simulink library "hmi"  (Simulink 8.1)
settings: Solver=ode1  StartTime=0.0  StopTime=Inf  FixedStep=0.001  RelTol=1e-3
PostLoadFcn:
  | , if any(exist('dsrtsu_mdlpostloadfcn', 'file') == [2, 3, 6]), try dsrtsu_mdlpostloadfcn('Execute', bdroot); catch fprintf('Error in PostLoadFcn (dsrtsu_mdlpostloadfcn) for model "%s":\n %s\n', bdroot, lasterr); end, end,
libraries: act x1, agg x1, brk x1, accs x1, ovr x1, otk x1, pkg x1, hcu_lib x1
settings Model: DSRTSU_INTERNAL_RTI_VER=450  DSRTSU_INTERNAL_RTI_TYPE=rti1401  RTICANMMDATA=struct('GeneralSetupData',struct('modelroot','D:\ELN150201_TAIWAN\trunk\AdasDragon\software\sw_development\arch\app\ifo','generalsettings',struct('filesettings',struct('destfolder',struct('Name','RTICANMM_FILES','Check',1),'buildfolder',struct('Name','.','Check',1),'AbsDestfolder',struct('Name','D:\ELN150201_TAIWAN\trunk\AdasDragon\software\sw_development\arch\app\ifo\RTICANMM_FILES'),'AbsBuildfolder',struct('Name','D:\ELN150201_TAIWAN\trunk\AdasDragon\software\sw_development\arch\app\ifo'))),'options',struct('addpaths',1,'rmpaths',1,'addtrcexclusion',logical(1),'cannavigator',struct('checkmonitoring',0),'show_usrtrc',0,'use_usrtrc',0),'advanced',struct('options',[1 1 1 1 1 1 1 1 1 1 1 1 1 1 1 1 1 1 1 1 1 1 1 1 1 1 1 1 1 1 1 1 1 1 1 1 1 1 1 1 1 1 1 1 1 1 1 1 1 1 1 1 1 1 1 1 1 1 1 1 1 1 1 1 1 1 1 1 1 1 1 1 1 1 1 1 1 1 1 1 1 1 1 1 1 1 1 1 1 1 1 1 1 1 1 1 1 1 1 1]),'MPSetup',{{}},'modelname','hmi','block','hmi'))  DSRTSU_INTERNAL_RTIFPGA=40  Creator=AT015411  LastModifiedBy=AT015555

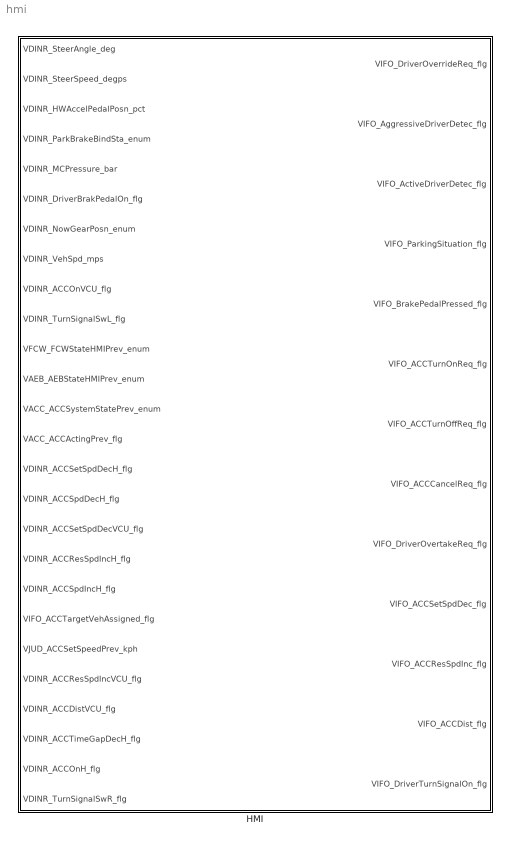
== system hmi ==
  HMI : Subsystem

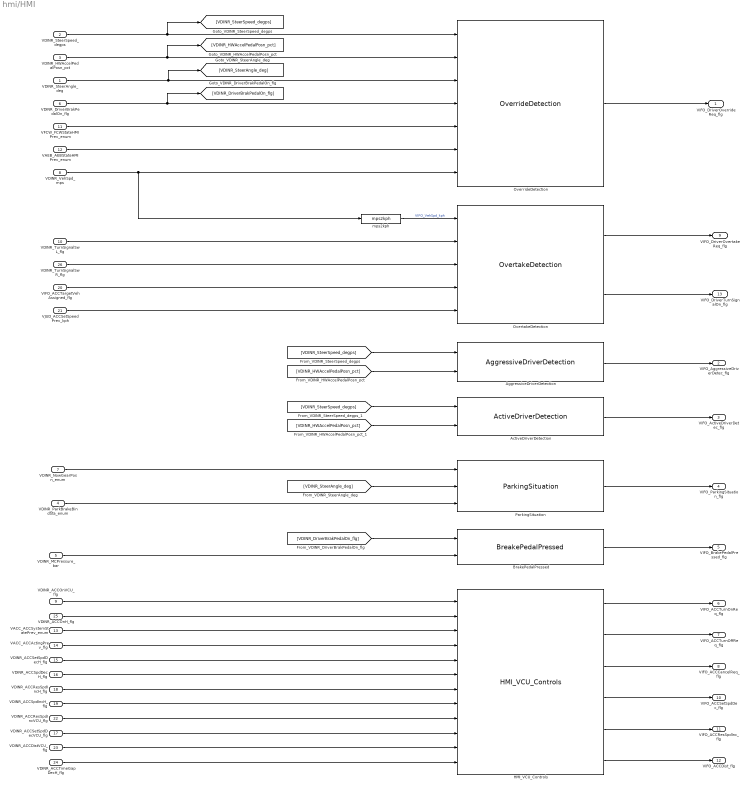
== system hmi/HMI ==
  VDINR_SteerAngle_deg : Inport
  VDINR_SteerSpeed_degps : Inport  Port=2
  VDINR_HWAccelPedalPosn_pct : Inport  Port=3
  VDINR_ParkBrakeBindSta_enum : Inport  Port=4
  VDINR_MCPressure_bar : Inport  Port=5
  VDINR_DriverBrakPedalOn_flg : Inport  Port=6
  VDINR_NowGearPosn_enum : Inport  Port=7
  VDINR_VehSpd_mps : Inport  Port=8
  VDINR_ACCOnVCU_flg : Inport  Port=9
  VDINR_TurnSignalSwL_flg : Inport  Port=10
  VFCW_FCWStateHMIPrev_enum : Inport  Port=11
  VAEB_AEBStateHMIPrev_enum : Inport  Port=12
  VACC_ACCSystemStatePrev_enum : Inport  Port=13
  VACC_ACCActingPrev_flg : Inport  Port=14
  VDINR_ACCSetSpdDecH_flg : Inport  Port=15
  VDINR_ACCSpdDecH_flg : Inport  Port=16
  VDINR_ACCSetSpdDecVCU_flg : Inport  Port=17
  VDINR_ACCResSpdIncH_flg : Inport  Port=18
  VDINR_ACCSpdIncH_flg : Inport  Port=19
  VIFO_ACCTargetVehAssigned_flg : Inport  Port=20
  VJUD_ACCSetSpeedPrev_kph : Inport  Port=21
  VDINR_ACCResSpdIncVCU_flg : Inport  Port=22
  VDINR_ACCDistVCU_flg : Inport  Port=23
  VDINR_ACCTimeGapDecH_flg : Inport  Port=24
  VDINR_ACCOnH_flg : Inport  Port=25
  VDINR_TurnSignalSwR_flg : Inport  Port=26
  ActiveDriverDetection : act/ActiveDriverDetection
  AggressiveDriverDetection : agg/AggressiveDriverDetection
  BrakePedalPressed : brk/BreakePedalPressed
  HMI_VCU_Controls : accs/HMI_VCU_Controls
  OverrideDetection : ovr/OverrideDetection
  OvertakeDetection : otk/OvertakeDetection
  ParkingSituation : pkg/ParkingSituation
  mps2kph : hcu_lib/mps2kph
  VIFO_DriverOverrideReq_flg : Outport
  VIFO_AggressiveDriverDetec_flg : Outport  Port=2
  VIFO_ActiveDriverDetec_flg : Outport  Port=3
  VIFO_ParkingSituation_flg : Outport  Port=4
  VIFO_BrakePedalPressed_flg : Outport  Port=5
  VIFO_ACCTurnOnReq_flg : Outport  Port=6
  VIFO_ACCTurnOffReq_flg : Outport  Port=7
  VIFO_ACCCancelReq_flg : Outport  Port=8
  VIFO_DriverOvertakeReq_flg : Outport  Port=9
  VIFO_ACCSetSpdDec_flg : Outport  Port=10
  VIFO_ACCResSpdInc_flg : Outport  Port=11
  VIFO_ACCDist_flg : Outport  Port=12
  VIFO_DriverTurnSignalOn_flg : Outport  Port=13
  wires:
  VDINR_ACCOnH_flg/1 -> HMI_VCU_Controls/2
  VDINR_ACCSpdIncH_flg/1 -> HMI_VCU_Controls/8
  VDINR_ACCSetSpdDecH_flg/1 -> HMI_VCU_Controls/5
  VDINR_ACCResSpdIncVCU_flg/1 -> HMI_VCU_Controls/9
  VDINR_ACCSpdDecH_flg/1 -> HMI_VCU_Controls/6
  VDINR_ACCResSpdIncH_flg/1 -> HMI_VCU_Controls/7
  VDINR_ACCSetSpdDecVCU_flg/1 -> HMI_VCU_Controls/10
  VDINR_ACCDistVCU_flg/1 -> HMI_VCU_Controls/11
  VDINR_ACCTimeGapDecH_flg/1 -> HMI_VCU_Controls/12
  HMI_VCU_Controls/6 -> VIFO_ACCDist_flg/1
  HMI_VCU_Controls/5 -> VIFO_ACCResSpdInc_flg/1
  HMI_VCU_Controls/4 -> VIFO_ACCSetSpdDec_flg/1
  VDINR_VehSpd_mps/1 -> mps2kph/1, OverrideDetection/7
  VDINR_SteerSpeed_degps/1 -> OverrideDetection/1, [VDINR_SteerSpeed_degps]
  VDINR_HWAccelPedalPosn_pct/1 -> [VDINR_HWAccelPedalPosn_pct], OverrideDetection/2
  VDINR_SteerAngle_deg/1 -> [VDINR_SteerAngle_deg], OverrideDetection/3
  VDINR_DriverBrakPedalOn_flg/1 -> OverrideDetection/4, [VDINR_DriverBrakPedalOn_flg]
  OverrideDetection/1 -> VIFO_DriverOverrideReq_flg/1
  AggressiveDriverDetection/1 -> VIFO_AggressiveDriverDetec_flg/1
  ActiveDriverDetection/1 -> VIFO_ActiveDriverDetec_flg/1
  VDINR_ParkBrakeBindSta_enum/1 -> ParkingSituation/3
  ParkingSituation/1 -> VIFO_ParkingSituation_flg/1
  [VDINR_DriverBrakPedalOn_flg] -> BrakePedalPressed/1
  VDINR_MCPressure_bar/1 -> BrakePedalPressed/2
  BrakePedalPressed/1 -> VIFO_BrakePedalPressed_flg/1
  VFCW_FCWStateHMIPrev_enum/1 -> OverrideDetection/5
  VAEB_AEBStateHMIPrev_enum/1 -> OverrideDetection/6
  [VDINR_SteerSpeed_degps] -> AggressiveDriverDetection/1
  [VDINR_SteerSpeed_degps] -> ActiveDriverDetection/1
  [VDINR_HWAccelPedalPosn_pct] -> AggressiveDriverDetection/2
  [VDINR_HWAccelPedalPosn_pct] -> ActiveDriverDetection/2
  [VDINR_SteerAngle_deg] -> ParkingSituation/2
  VDINR_NowGearPosn_enum/1 -> ParkingSituation/1
  HMI_VCU_Controls/1 -> VIFO_ACCTurnOnReq_flg/1
  HMI_VCU_Controls/2 -> VIFO_ACCTurnOffReq_flg/1
  HMI_VCU_Controls/3 -> VIFO_ACCCancelReq_flg/1
  VDINR_ACCOnVCU_flg/1 -> HMI_VCU_Controls/1
  VACC_ACCSystemStatePrev_enum/1 -> HMI_VCU_Controls/3
  VACC_ACCActingPrev_flg/1 -> HMI_VCU_Controls/4
  VDINR_TurnSignalSwL_flg/1 -> OvertakeDetection/2
  VIFO_ACCTargetVehAssigned_flg/1 -> OvertakeDetection/4
  mps2kph/1 -> OvertakeDetection/1  "VIFO_VehSpd_kph"
  OvertakeDetection/1 -> VIFO_DriverOvertakeReq_flg/1
  VJUD_ACCSetSpeedPrev_kph/1 -> OvertakeDetection/5
  VDINR_TurnSignalSwR_flg/1 -> OvertakeDetection/3
  OvertakeDetection/2 -> VIFO_DriverTurnSignalOn_flg/1
